simulink library "dspxfrm3"  (Simulink 8.3)
settings: Solver=ode45  SolverMode=SingleTasking  StartTime=0.0  StopTime=10.0  RelTol=1e-3
values from neighbouring files (symbols this model uses):
  D = D + B    [rebuffer_delay.m]
undefined symbols (not defined in the file or in its folder): dfilt, magnitude, Rows
libraries: dspsigops x6, dspxfrm3 x6, dspmtrx3 x6, dspsigattribs x5, dspmlti4 x2, dsparch4 x1, dspspect3 x1
settings Model: RequirementInfo=9  FPTRunName=Active  Creator=szlotkin  LastModifiedBy=apakyari  CovMetricSettings=d  ExtModeAutoUpdateStatusClock=off

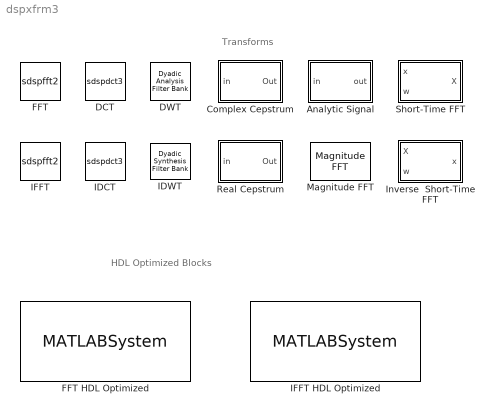
== system dspxfrm3 ==
  note: Transforms
  note: HDL Optimized Blocks
  Analytic Signal : Subsystem  mask(Analytic Signal){N=100, InputProcessing=Columns as channels (frame based)}
      mask prompts: N "Filter order (must be even):"; InputProcessing "Input processing:"
      mask help: Complex analytic signal of input.
      mask init:
      | x = [0,NaN,100,NaN,[58 58],NaN,[24 92],NaN,[58 24 24 58],NaN,[58 64 68 72 76 80 84 88],NaN, [42 42],NaN,[8 76],NaN,[72 68 64 60 56 52 48 42 36 32 28 24 20 16 12],NaN,[32 43 45 43 35]];
      | y = [0,NaN,100,NaN,[43 8],NaN,[16 16],NaN,[18 18 17 17],NaN,[16 24 36 24 28 28 32 16],NaN, [92 56],NaN,[64 64],NaN,[64 80 76 76 72 84 72 64 72 84 72 76 76 80 64],NaN,[51 33 41 33 35] ];
      | b=dspblkanalytic2('design',true,N);
      | dspblkanalytic2('setup',true,InputProcessing);
      mask Help: eval('blocksethelp');
      mask TypeOptions InputProcessing: Columns as channels (frame based) | Elements as channels (sample based) | Inherited (this choice will be removed - see release notes)
      mask Display: plot(x,y)
  Complex Cepstrum : Subsystem  mask(Complex Cepstrum){inheritFFT=on, N=64}
      mask prompts: inheritFFT "Inherit FFT length from input port dimensions"; N "FFT length:"
      mask help: Complex cepstrum of input signal. Input is modified to remove possible phase discontinuity at +/- pi radians.
      mask init:
      | dspblkceps('init');
      mask Help: eval('blocksethelp');
      mask Callback inheritFFT: dspblkceps
      mask Display: disp('Complex\n Cepstrum')
  DCT : S-Function  DialogController=dvDDGCreate  DialogControllerArgs=DataTag4  FunctionName=sdspdct3  Parameters=0, CompMethod,Dimension, 1, 0, 0, 0,1,outputMin,outputMax,dtInfo.firstCoeffMode,dtInfo.firstCoeffWordLength,dtInfo.firstCoeffFracLength,dtInfo.prodOutputMode,dtInfo.prodOutputWordLength,dtInfo.prodOutputFracLength,dtInfo.accumMode,dtInfo.accumWordLength,dtInfo.accumFracLength,dtInfo.outputMode,dtInfo.outputWordLength,dtInfo.outputFracLength,dtInfo.roundingMode,dtInfo.overflowMode  EnableBusSupport=on  mask(DCT){CompMethod=Table lookup, Dimension=0, TableOpt=Speed, BitRevOrder=off, SkipNorm=off, firstCoeffMode=Same word length as input, firstCoeffWordLength=16, firstCoeffFracLength=15, firstCoeffDataTypeStr=Inherit: Same word length as input, firstCoeffLastDataTypeStr=Inherit: Same word length as input, outputMode=Inherit via internal rule, outputWordLength=16, outputFracLength=15, outputDataTypeStr=Inherit: Inherit via internal rule, outputLastDataTypeStr=Inherit: Inherit via internal rule, outputMin=[], outputMax=[], accumMode=Inherit via internal rule, accumWordLength=32, accumFracLength=30, accumDataTypeStr=Inherit: Inherit via internal rule, accumLastDataTypeStr=Inherit: Inherit via internal rule, prodOutputMode=Inherit via internal rule, prodOutputWordLength=32, prodOutputFracLength=30, prodOutputDataTypeStr=Inherit: Inherit via internal rule, prodOutputLastDataTypeStr=Inherit: Inherit via internal rule, roundingMode=Floor, overflowMode=off, LockScale=off}
      mask prompts: CompMethod "Sine and cosine computation:"; TableOpt "Optimize twiddle table for:"; BitRevOrder "Output in bit-reversed order"; SkipNorm "Skip divide-by-two on butterfly outputs for fixed-point signals"; firstCoeffMode "Fixed-point sine table attributes:"; firstCoeffWordLength "Sine table word length:"; firstCoeffFracLength "Sine table fraction length:"; firstCoeffDataTypeStr "Sine table data type string:"; firstCoeffLastDataTypeStr "Last sine table data type string:"; outputMode "Fixed-point output attributes:"; outputWordLength "Output word length:"; outputFracLength "Output fraction length:"; outputDataTypeStr "Output data type string:"; outputLastDataTypeStr "Last output data type string:"; outputMin "Output minimum:"; outputMax "Output maximum:"; accumMode "Fixed-point accumulator attributes:"; accumWordLength "Accumulator word length:"; accumFracLength "Accumulator fraction length:"; accumDataTypeStr "Accum data type string:"; accumLastDataTypeStr "Last accum data type string:"; prodOutputMode "Fixed-point product output attributes:"; prodOutputWordLength "Product output word length:"; prodOutputFracLength "Product output fraction length:"; prodOutputDataTypeStr "ProdOutput data type string:"; prodOutputLastDataTypeStr "Last prodOutput data type string:"; roundingMode "Round integer calculations toward:"; overflowMode "Saturate on integer overflow"; LockScale "Lock scaling"
      mask help: Compute the discrete cosine transform (DCT) across the first dimension of the input. The first dimension of the input must have a power-of-two length.
      mask init:
      | Dimension = 1;
      | blkh   = gcbh;
      | dtRows = dspblkGetFFTDTRowInfo();
      | dtInfo = dspGetUDTFixptDataTypeInfo(blkh, dtRows, true);
      mask Help: eval('blocksethelp');
      mask TypeOptions CompMethod: Trigonometric fcn | Table lookup
      mask TypeOptions TableOpt: Speed | Memory
      mask TypeOptions firstCoeffMode: Same word length as input | Specify word length
      mask TypeOptions outputMode: Inherit via internal rule | Same as input | Binary point scaling | Slope and bias scaling
      mask TypeOptions accumMode: Inherit via internal rule | Same as product output | Same as input | Binary point scaling | Slope and bias scaling
      mask TypeOptions prodOutputMode: Inherit via internal rule | Same as input | Binary point scaling | Slope and bias scaling
      mask TypeOptions roundingMode: Ceiling | Convergent | Floor | Nearest | Round | Simplest | Zero
      mask Display: disp(' DCT')
  DWT : dspmlti4/Dyadic Analysis Filter Bank  Wname=User-defined  OrdRec_ordDec=[1 / 1]  Order=2  LPF="[0.0352   -0.0854   -0.1350   0.4599   0.8069   0.3327]"  HPF="[-0.3327    0.8069   -0.4599   -0.1350    0.0854    0.0352]"  NumLevels=2  tree=Symmetric  Output=Single port
  FFT : S-Function  DialogController=dspDDGCreate  DialogControllerArgs=DataTag5  FunctionName=sdspfft2  Parameters=0,2,TableOpt,1,BitRevOrder,0,SkipNorm,0,InheritFFTLength,FFTLength,WrapInput,1,outputMin,outputMax,RowConvenienceOn,plannerMethod,FFTImplementation,dtInfo.firstCoeffMode,dtInfo.firstCoeffWordLength,dtInfo.firstCoeffFracLength,dtInfo.prodOutputMode,dtInfo.prodOutputWordLength,dtInfo.prodOutputFracLength,dtInfo.accumMode,dtInfo.accumWordLength,dtInfo.accumFracLength,dtInfo.outputMode,dtInfo.outputWordLength,dtInfo.outputFracLength,dtInfo.roundingMode,dtInfo.overflowMode  EnableBusSupport=off  mask(FFT){CompMethod=Table lookup, TableOpt=NEW, TableOptActive=Speed, BitRevOrder=off, InheritFFTLength=on, FFTLength=64, WrapInput=on, RowConvenienceOn=on, FFTImplementation=Auto, additionalParams=off, SkipNorm=off, allowOverrides=on, firstCoeffMode=Same word length as input, firstCoeffWordLength=16, firstCoeffFracLength=15, firstCoeffDataTypeStr=Inherit: Same word length as input, firstCoeffLastDataTypeStr=Inherit: Same word length as input, outputMode=Inherit via internal rule, outputWordLength=16, outputFracLength=15, outputDataTypeStr=Inherit: Inherit via internal rule, outputLastDataTypeStr=Inherit: Inherit via internal rule, outputMin=[], outputMax=[], accumMode=Inherit via internal rule, accumWordLength=32, accumFracLength=30, accumDataTypeStr=Inherit: Inherit via internal rule, accumLastDataTypeStr=Inherit: Inherit via internal rule, prodOutputMode=Inherit via internal rule, prodOutputWordLength=32, prodOutputFracLength=30, prodOutputDataTypeStr=Inherit: Inherit via internal rule, prodOutputLastDataTypeStr=Inherit: Inherit via internal rule, roundingMode=Floor, overflowMode=off, LockScale=off}
      mask prompts: CompMethod "Twiddle factor computation:"; TableOpt "Optimize table for (obsolete):"; TableOptActive "Optimize table for:"; BitRevOrder "Output in bit-reversed order"; InheritFFTLength "Inherit FFT length from input dimensions"; FFTLength "FFT length:"; WrapInput "Wrap input data when FFT length is shorter than input length"; RowConvenienceOn "Perform row convenience"; FFTImplementation "FFT implementation:"; additionalParams "---------- Show additional parameters ----------"; SkipNorm "Skip divide-by-two on butterfly outputs for fixed-point signals"; allowOverrides "Allow overrides from DSP Fixed-Point Attributes blocks"; firstCoeffMode "Fixed-point sine table attributes:"; firstCoeffWordLength "Sine table word length:"; firstCoeffFracLength "Sine table fraction length:"; firstCoeffDataTypeStr "Sine table data type string:"; firstCoeffLastDataTypeStr "Last sine table data type string:"; outputMode "Fixed-point output attributes:"; outputWordLength "Output word length:"; outputFracLength "Output fraction length:"; outputDataTypeStr "Output data type string:"; outputLastDataTypeStr "Last output data type string:"; outputMin "Output minimum:"; outputMax "Output maximum:"; accumMode "Fixed-point accumulator attributes:"; accumWordLength "Accumulator word length:"; accumFracLength "Accumulator fraction length:"; accumDataTypeStr "Accum data type string:"; accumLastDataTypeStr "Last accum data type string:"; prodOutputMode "Fixed-point product output attributes:"; prodOutputWordLength "Product output word length:"; prodOutputFracLength "Product output fraction length:"; prodOutputDataTypeStr "ProdOutput data type string:"; prodOutputLastDataTypeStr "Last prodOutput data type string:"; roundingMode "Round integer calculations toward:"; overflowMode "Saturate on integer overflow"; LockScale "Lock scaling"
      mask help:
      | Compute the fast Fourier transform (FFT) across the first dimension of the input.
      |
      | When you set the 'FFT implementation' parameter to 'Radix-2', the FFT length must be a power of two.
      mask init:
      | blkh = gcbh;
      | plannerMethod = dspfftcontrol();
      | if ~(strcmp(get_param(blkh,'TableOpt'),'HYBRID') ||  strcmp(get_param(blkh,'TableOpt'),'NEW'))
      |   % this block lives in older version of SP BlockSet
      |     set_param(blkh,'TableOptActive',get_param(blkh,'TableOpt'));
      |     set_param(blkh,'TableOpt','HYBRID');
      |     if (strcmp(get_param(blkh,'SkipNorm'),'on'))
      |         set_param(blkh,'SkipNorm','off');
      |     else
      |         set_param(blkh,'SkipNorm','on');
      |     end
      | end
      | dtRows = dspblkGetFFTDTRowInfo();
      | dtInfo = dspGetUDTFixptDataTypeInfo(blkh, dtRows, true);
      mask Help: eval('blocksethelp');
      mask TypeOptions CompMethod: Trigonometric fcn | Table lookup
      mask TypeOptions TableOpt: Speed | Memory | HYBRID | NEW
      mask TypeOptions TableOptActive: Speed | Memory
      mask TypeOptions FFTImplementation: Auto | Radix-2 | FFTW
      mask TypeOptions firstCoeffMode: Same word length as input | Specify word length | Same as input | Same as output | User-defined | Binary point scaling | Slope and bias scaling
      mask TypeOptions outputMode: Inherit via internal rule | Same as input | Binary point scaling | Slope and bias scaling | User-defined
      mask TypeOptions accumMode: Inherit via internal rule | Same as product output | Same as input | Binary point scaling | Slope and bias scaling | User-defined
      mask TypeOptions prodOutputMode: Inherit via internal rule | Same as input | Binary point scaling | Slope and bias scaling | User-defined
      mask TypeOptions roundingMode: Ceiling | Convergent | Floor | Nearest | Round | Simplest | Zero
      mask Display: disp('  FFT ');
  FFT HDL Optimized : MATLABSystem  System=dsp.HDLFFT  Normalize=off  FFTLengthSource=Property  FFTLength=1024  RoundingMethod=Floor  OverflowAction=Wrap  ValidInputPort=on  StartOutputPort=off  EndOutputPort=off
      mask Type: dsp.HDLFFT
      mask Display:
      | disp(['FFT' char(10) 'HDL Optimized' char(10) 'Latency, 1589']);
      | port_label('input',1,'dataIn');
      | port_label('input',2,'validIn');
      | port_label('output',1,'dataOut');
      | port_label('output',2,'validOut');
  IDCT : S-Function  DialogController=dvDDGCreate  DialogControllerArgs=DataTag6  FunctionName=sdspdct3  Parameters=1,CompMethodActive, Dimension, 1, 0, 0, 0,outSamplingMode,outputMin,outputMax,dtInfo.firstCoeffMode,dtInfo.firstCoeffWordLength,dtInfo.firstCoeffFracLength,dtInfo.prodOutputMode,dtInfo.prodOutputWordLength,dtInfo.prodOutputFracLength,dtInfo.accumMode,dtInfo.accumWordLength,dtInfo.accumFracLength,dtInfo.outputMode,dtInfo.outputWordLength,dtInfo.outputFracLength,dtInfo.roundingMode,dtInfo.overflowMode  EnableBusSupport=on  mask(IDCT){CompMethod=HYBRID, CompMethodActive=Table lookup, Dimension=0, TableOpt=Speed, BitRevOrder=off, outSamplingMode=Sample based, SkipNorm=off, firstCoeffMode=Same word length as input, firstCoeffWordLength=16, firstCoeffFracLength=15, firstCoeffDataTypeStr=Inherit: Same word length as input, firstCoeffLastDataTypeStr=Inherit: Same word length as input, outputMode=Inherit via internal rule, outputWordLength=16, outputFracLength=15, outputDataTypeStr=Inherit: Inherit via internal rule, outputLastDataTypeStr=Inherit: Inherit via internal rule, outputMin=[], outputMax=[], accumMode=Inherit via internal rule, accumWordLength=32, accumFracLength=30, accumDataTypeStr=Inherit: Inherit via internal rule, accumLastDataTypeStr=Inherit: Inherit via internal rule, prodOutputMode=Inherit via internal rule, prodOutputWordLength=32, prodOutputFracLength=30, prodOutputDataTypeStr=Inherit: Inherit via internal rule, prodOutputLastDataTypeStr=Inherit: Inherit via internal rule, roundingMode=Floor, overflowMode=off, LockScale=off}
      mask prompts: CompMethod "Twiddle factor computation obsolete:"; CompMethodActive "Sine and cosine computation:"; TableOpt "Optimize twiddle table for:"; BitRevOrder "Output in bit-reversed order"; outSamplingMode "OUtput sampling mode"; SkipNorm "Skip divide-by-two on butterfly outputs for fixed-point signals"; firstCoeffMode "Fixed-point sine table attributes:"; firstCoeffWordLength "Sine table word length:"; firstCoeffFracLength "Sine table fraction length:"; firstCoeffDataTypeStr "Sine table data type string:"; firstCoeffLastDataTypeStr "Last sine table data type string:"; outputMode "Fixed-point output attributes:"; outputWordLength "Output word length:"; outputFracLength "Output fraction length:"; outputDataTypeStr "Output data type string:"; outputLastDataTypeStr "Last output data type string:"; outputMin "Output minimum:"; outputMax "Output maximum:"; accumMode "Fixed-point accumulator attributes:"; accumWordLength "Accumulator word length:"; accumFracLength "Accumulator fraction length:"; accumDataTypeStr "Accum data type string:"; accumLastDataTypeStr "Last accum data type string:"; prodOutputMode "Fixed-point product output attributes:"; prodOutputWordLength "Product output word length:"; prodOutputFracLength "Product output fraction length:"; prodOutputDataTypeStr "ProdOutput data type string:"; prodOutputLastDataTypeStr "Last prodOutput data type string:"; roundingMode "Round integer calculations toward:"; overflowMode "Saturate on integer overflow"; LockScale "Lock scaling"
      mask help: Compute the inverse discrete cosine transform (IDCT) across the first dimension of the input. The first dimension of the input must have a power-of-two length.
      mask init:
      | Dimension = 1;
      | blkh      = gcbh;
      | if ~(strcmp(get_param(blkh,'CompMethod'),'HYBRID') ||  strcmp(get_param(blkh,'CompMethod'),'NEW'))
      |   % this block lives in older version of SP BlockSet
      |     set_param(blkh,'outSamplingMode','Frame based');
      |     set_param(blkh,'CompMethodActive',get_param(blkh,'CompMethod'));
      |     set_param(blkh,'CompMethod','HYBRID');
      | end
      | dtRows = dspblkGetFFTDTRowInfo();
      | dtInfo = dspGetUDTFixptDataTypeInfo(blkh, dtRows, true);
      mask Help: eval('blocksethelp');
      mask TypeOptions CompMethod: Trigonometric fcn | Table lookup | HYBRID | NEW
      mask TypeOptions CompMethodActive: Trigonometric fcn | Table lookup
      mask TypeOptions TableOpt: Speed | Memory
      mask TypeOptions outSamplingMode: Sample based | Frame based
      mask TypeOptions firstCoeffMode: Same word length as input | Specify word length
      mask TypeOptions outputMode: Inherit via internal rule | Same as input | Binary point scaling | Slope and bias scaling
      mask TypeOptions accumMode: Inherit via internal rule | Same as product output | Same as input | Binary point scaling | Slope and bias scaling
      mask TypeOptions prodOutputMode: Inherit via internal rule | Same as input | Binary point scaling | Slope and bias scaling
      mask TypeOptions roundingMode: Ceiling | Convergent | Floor | Nearest | Round | Simplest | Zero
      mask Display: disp('IDCT')
  IDWT : dspmlti4/Dyadic Synthesis Filter Bank  Wname=User-defined  OrdRec_ordDec=[1 / 1]  Order=2  LPF="[0.3327    0.8069    0.4599   -0.1350   -0.0854    0.0352]"  HPF="[0.0352    0.0854   -0.1350   -0.4599    0.8069   -0.3327]"  NumLevels=2  tree=Symmetric  Input=Single port
  IFFT : S-Function  DialogController=dspDDGCreate  DialogControllerArgs=DataTag7  FunctionName=sdspfft2  Parameters=1,2,TableOpt,1,BitRevOrder,cs_in,SkipNorm,0,InheritFFTLength,FFTLength,WrapInput,outSamplingMode,outputMin,outputMax,RowConvenienceOn,plannerMethod,FFTImplementation,dtInfo.firstCoeffMode,dtInfo.firstCoeffWordLength,dtInfo.firstCoeffFracLength,dtInfo.prodOutputMode,dtInfo.prodOutputWordLength,dtInfo.prodOutputFracLength,dtInfo.accumMode,dtInfo.accumWordLength,dtInfo.accumFracLength,dtInfo.outputMode,dtInfo.outputWordLength,dtInfo.outputFracLength,dtInfo.roundingMode,dtInfo.overflowMode  EnableBusSupport=off  mask(IFFT){CompMethod=Table lookup, TableOpt=NEW, TableOptActive=Speed, BitRevOrder=off, cs_in=off, SkipNorm=on, InheritFFTLength=on, FFTLength=64, WrapInput=on, mode=Complex, outSamplingMode=Sample based, RowConvenienceOn=on, FFTImplementation=Auto, additionalParams=off, allowOverrides=on, firstCoeffMode=Same word length as input, firstCoeffWordLength=16, firstCoeffFracLength=15, firstCoeffDataTypeStr=Inherit: Same word length as input, firstCoeffLastDataTypeStr=Inherit: Same word length as input, outputMode=Inherit via internal rule, outputWordLength=16, outputFracLength=15, outputDataTypeStr=Inherit: Inherit via internal rule, outputLastDataTypeStr=Inherit: Inherit via internal rule, outputMin=[], outputMax=[], accumMode=Inherit via internal rule, accumWordLength=32, accumFracLength=30, accumDataTypeStr=Inherit: Inherit via internal rule, accumLastDataTypeStr=Inherit: Inherit via internal rule, prodOutputMode=Inherit via internal rule, prodOutputWordLength=32, prodOutputFracLength=30, prodOutputDataTypeStr=Inherit: Inherit via internal rule, prodOutputLastDataTypeStr=Inherit: Inherit via internal rule, roundingMode=Floor, overflowMode=off, LockScale=off}
      mask prompts: CompMethod "Twiddle factor computation:"; TableOpt "Optimize table for (obsolete):"; TableOptActive "Optimize table for:"; BitRevOrder "Input is in bit-reversed order"; cs_in "Input is conjugate symmetric"; SkipNorm "Skip scaling"; InheritFFTLength "Inherit FFT length from input dimensions"; FFTLength "FFT length:"; WrapInput "Wrap input data when FFT length is shorter than input length"; mode "Output:"; outSamplingMode "OUtput sampling mode"; RowConvenienceOn "Perform row convenience"; FFTImplementation "FFT implementation:"; additionalParams "---------- Show additional parameters ----------"; allowOverrides "Allow overrides from DSP FPA Fixed-Point Attributes blocks"; firstCoeffMode "Fixed-point sine table attributes:"; firstCoeffWordLength "Sine table word length:"; firstCoeffFracLength "Sine table fraction length:"; firstCoeffDataTypeStr "Sine table data type string:"; firstCoeffLastDataTypeStr "Last sine table data type string:"; outputMode "Fixed-point output attributes:"; outputWordLength "Output word length:"; outputFracLength "Output fraction length:"; outputDataTypeStr "Output data type string:"; outputLastDataTypeStr "Last output data type string:"; outputMin "Output minimum:"; outputMax "Output maximum:"; accumMode "Fixed-point accumulator attributes:"; accumWordLength "Accumulator word length:"; accumFracLength "Accumulator fraction length:"; accumDataTypeStr "Accum data type string:"; accumLastDataTypeStr "Last accum data type string:"; prodOutputMode "Fixed-point product output attributes:"; prodOutputWordLength "Product output word length:"; prodOutputFracLength "Product output fraction length:"; prodOutputDataTypeStr "ProdOutput data type string:"; prodOutputLastDataTypeStr "Last prodOutput data type string:"; roundingMode "Round integer calculations toward:"; overflowMode "Saturate on integer overflow"; LockScale "Lock scaling"
      mask help:
      | Compute the inverse fast Fourier transform (IFFT) across the first dimension of the input.
      |
      | When you set the 'FFT implementation' parameter to 'Radix-2', the FFT length must be a power of two.
      mask init:
      | blkh = gcbh;
      | plannerMethod = dspfftcontrol();
      | if ~(strcmp(get_param(blkh,'TableOpt'),'HYBRID') ||  strcmp(get_param(blkh,'TableOpt'),'NEW'))
      |   % this block lives in older version of SP BlockSet
      | %     set_param(blkh,'frameSpecViaDialog','off');
      |     set_param(blkh,'outSamplingMode','Frame based');
      |     set_param(blkh,'TableOptActive',get_param(blkh,'TableOpt'));
      |     set_param(blkh,'TableOpt','HYBRID');
      |     if (strcmp(get_param(blkh,'SkipNorm'),'on'))
      |         set_param(blkh,'SkipNorm','off');
      |     else
      |         set_param(blkh,'SkipNorm','on');
      |     end    
      | end
      | dtRows = dspblkGetFFTDTRowInfo();
      | dtInfo = dspGetUDTFixptDataTypeInfo(blkh, dtRows, true);
      mask Help: eval('blocksethelp');
      mask TypeOptions CompMethod: Trigonometric fcn | Table lookup
      mask TypeOptions TableOpt: Speed | Memory | HYBRID | NEW
      mask TypeOptions TableOptActive: Speed | Memory
      mask TypeOptions mode: Real | Complex
      mask TypeOptions outSamplingMode: Sample based | Frame based
      mask TypeOptions FFTImplementation: Auto | Radix-2 | FFTW
      mask TypeOptions firstCoeffMode: Same word length as input | Specify word length | Same as input | Same as output | User-defined | Binary point scaling | Slope and bias scaling
      mask TypeOptions outputMode: Inherit via internal rule | Same as input | Binary point scaling | Slope and bias scaling | User-defined
      mask TypeOptions accumMode: Inherit via internal rule | Same as product output | Same as input | Binary point scaling | Slope and bias scaling | User-defined
      mask TypeOptions prodOutputMode: Inherit via internal rule | Same as input | Binary point scaling | Slope and bias scaling | User-defined
      mask TypeOptions roundingMode: Ceiling | Convergent | Floor | Nearest | Round | Simplest | Zero
      mask Display: disp('  IFFT')
  IFFT HDL Optimized : MATLABSystem  System=dsp.HDLIFFT  Normalize=on  FFTLengthSource=Property  FFTLength=1024  RoundingMethod=Floor  OverflowAction=Wrap  ValidInputPort=on  StartOutputPort=off  EndOutputPort=off
      mask Type: dsp.HDLIFFT
      mask Display:
      | disp(['IFFT' char(10) 'HDL Optimized' char(10) 'Latency, 1589']);
      | port_label('input',1,'dataIn');
      | port_label('input',2,'validIn');
      | port_label('output',1,'dataOut');
      | port_label('output',2,'validOut');
  Inverse  Short-Time FFT : Subsystem  mask(Inverse Short-Time FFT){W=512, OvLap=384, OutFrameSize=512, InConjSymm=on, DoAssert=off, Tol=1e-4}
      mask prompts: W "Analysis window length:"; OvLap "Overlap between consecutive STFFT frames (in samples):"; OutFrameSize "Samples per output frame:"; InConjSymm "Input is conjugate symmetric"; DoAssert "Assert if analysis window does not support perfect signal reconstruction"; Tol "Reconstruction error tolerance:"
      mask help:
      | Reconstructs a signal from its Short-Time FFT (STFFT) by using the OLA method. The block takes as an input the analysis window w[n] used in the generation of the STFFT to normalize the output signal.
      |
      | Optionally, the block asserts if the analysis window does not satisfy constraints that permit perfect reconstruction of the signal.
      mask init:
      | L = dspblkistfft('init',DoAssert,OvLap,W,InConjSymm);
      mask Help: eval('blocksethelp');
      mask Callback DoAssert: dspblkistfft('dynamic');
      mask Display:
      | port_label('input',1,'X[nL,k]')
      | port_label('output',1,'x[n]')
      | port_label('input',2,'w[n]')
  Magnitude FFT : dspspect3/Magnitude FFT  mag_or_magsq=Magnitude squared  FFTImplementation=Auto  fftLenInherit=off  fftsize=256  WrapInput=on
  Real Cepstrum : Subsystem  mask(Real Cepstrum){inheritFFT=on, N=64}
      mask prompts: inheritFFT "Inherit FFT length from input port dimensions"; N "FFT length:"
      mask help: Real cepstrum of input signal.
      mask init:
      | dspblkceps('init');
      mask Help: eval('blocksethelp');
      mask Callback inheritFFT: dspblkceps
      mask Display: disp('Real\nCepstrum')
  Short-Time FFT : Subsystem  mask(Short-Time FFT){W=512, OvLap=384, M=1024, TreatMby1Signals=One channel}
      mask prompts: W "Analysis window length:"; OvLap "Overlap between consecutive windows (in samples):"; M "FFT length:"; TreatMby1Signals "Treat Mx1 and unoriented sample-based signals as:"
      mask help:
      | Output the Short-Time FFT of the input signal x[n].
      | Uses an externally specified analysis window w[n].
      mask init:
      | dspSetFrameUpgradeParameter(gcbh, 'TreatMby1Signals', 'M channels (this choice will be removed - see release notes)');
      | 
      | if W == 1
      |     error('spblockset:ShortTimeFFT:winLenOne', ...
      |           'The analysis window length must be greater than 1');
      | end
      | 
      | L = W-OvLap;
      | BufferBlkName = [gcb '/Rebuffer'];
      | set_param(BufferBlkName, 'TreatMby1Signals', ...
      |           get_param(gcb, 'TreatMby1Signals'));
      mask Help: eval('blocksethelp');
      mask TypeOptions TreatMby1Signals: One channel | M channels (this choice will be removed - see release notes)
      mask Display:
      | port_label('input',1,'x[n]')
      | port_label('input',2,'w[n]')
      | port_label('output',1,'X[nL,k]')

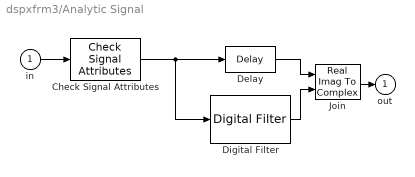
== system dspxfrm3/Analytic Signal ==
  in : Inport
  Check Signal Attributes : dspsigattribs/Check Signal Attributes  SystemSampleTime=-1  SigAttribCheckMethod=Does not match attributes exactly  Complexity=Ignore  Frame=Ignore  DimsCheckMethod=Ignore  Dimensions=1-D  DatatypeCheckMethod=Is...  DatatypeGeneral=Floating-point  DtypeFloatSpecific=Any floating-point  DtypeFixedSpecific=Any fixed-point  DtypeIntSpecific=Any integer  SampleMode=Ignore
  Delay : dspsigops/Delay  InputProcessing=Columns as channels (frame based)  dly_unit=Samples  delay=N/2  ic_detail=off  dif_ic_for_ch=off  dif_ic_for_dly=off  ic=0  reset_popup=None
  Digital Filter : dsparch4/Digital Filter  TypePopup=FIR (all zeros)  IIRFiltStruct=Direct form II transposed  AllPoleFiltStruct=Direct form  FIRFiltStruct=Direct form transposed  CoeffSource=Specify via dialog  NumCoeffs=b  DenCoeffs=[1 0.1]  BiQuadCoeffs=[1 0.3 0.4 1 0.1 0.2]  LatticeCoeffs=[0.2 0.4]  denIgnore=on  FiltPerSampPopup=One filter per frame  IC=0  ICnum=0  ICden=0  roundingMode=Floor  overflowMode=off  ScaleValues=1  scaleValueFracLength=14  stageInFracLength=15  stageOutFracLength=15  FilterSource=Specify via dialog  dfiltObjectName=dfilt.dffir([1 2 1])  InputProcessing=Columns as channels (frame based)
  Join : RealImagToComplex
  out : Outport  InitialOutput=0
  wires:
  Check Signal Attributes/1 -> Digital Filter/1, Delay/1
  in/1 -> Check Signal Attributes/1
  Join/1 -> out/1
  Delay/1 -> Join/1
  Digital Filter/1 -> Join/2

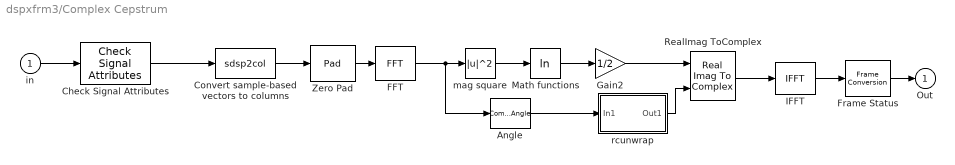
== system dspxfrm3/Complex Cepstrum ==
  in : Inport
  Angle : ComplexToMagnitudeAngle  Output=Angle
  Check Signal Attributes : dspsigattribs/Check Signal Attributes  SigAttribCheckMethod=Does not match attributes exactly  Complexity=Real  Frame=Ignore  DimsCheckMethod=Ignore  Dimensions=1-D  DatatypeCheckMethod=Is...  DatatypeGeneral=Floating-point  DtypeFloatSpecific=Any floating-point  DtypeFixedSpecific=Any fixed-point  DtypeIntSpecific=Any integer  SampleMode=Discrete
  Convert sample-based vectors to columns : S-Function  FunctionName=sdsp2col  EnableBusSupport=off
  FFT : dspxfrm3/FFT  CompMethod=Table lookup  TableOpt=NEW  TableOptActive=Speed  BitRevOrder=off  InheritFFTLength=on  FFTLength=64  RowConvenienceOn=on  FFTImplementation=Auto  SkipNorm=off  firstCoeffDataTypeStr=Inherit: Same word length as input  firstCoeffLastDataTypeStr=Inherit: Same word length as input  outputMin=[]  outputMax=[]  roundingMode=Floor  overflowMode=off
  Frame Status : FrameConversion  OutFrame=Sample-based
  Gain2 : Gain  Gain=1/2  SaturateOnIntegerOverflow=on  OutDataTypeStr=Inherit: Same as input  ParamDataTypeStr=Inherit: Same as input
  IFFT : dspxfrm3/IFFT  CompMethod=Table lookup  TableOpt=HYBRID  TableOptActive=Speed  BitRevOrder=off  cs_in=on  SkipNorm=on  InheritFFTLength=on  FFTLength=64  mode=Real  outSamplingMode=Frame based  RowConvenienceOn=on  FFTImplementation=Auto  firstCoeffDataTypeStr=Inherit: Same word length as input  firstCoeffLastDataTypeStr=Inherit: Same word length as input  outputMin=[]  outputMax=[]  roundingMode=Floor  overflowMode=off
  Math functions : Math  Operator=log  SaturateOnIntegerOverflow=on
  RealImag ToComplex : RealImagToComplex
  Zero Pad : dspsigops/Pad  padAlong=None  dimsToPad=1  valSrc=Specify via dialog  padVal=0  spec=Output size  padNumOutRowsSpecMethod=User-specified  numOutRows=N  padNumOutColsSpecMethod=User-specified  numOutCols=1  isVarDimsMode=off  padBeginning=0  padEnd=0  outSizeMode=User-specified  outSize=1  padSigAt=End  trunc_flag=None  roundingMode=Floor  overflowMode=off  truncOrWrapMode=Truncate  wrap_flag=None
  mag square : Math  Operator=magnitude^2  SaturateOnIntegerOverflow=on
  rcunwrap : Subsystem
  Out : Outport  InitialOutput=0
  wires:
  Check Signal Attributes/1 -> Convert sample-based vectors to columns/1
  RealImag ToComplex/1 -> IFFT/1
  Frame Status/1 -> Out/1
  Zero Pad/1 -> FFT/1
  Convert sample-based vectors to columns/1 -> Zero Pad/1
  IFFT/1 -> Frame Status/1
  Angle/1 -> rcunwrap/1(In1)
  FFT/1 -> Angle/1, mag square/1
  in/1 -> Check Signal Attributes/1
  Math functions/1 -> Gain2/1
  mag square/1 -> Math functions/1
  rcunwrap/1(Out1) -> RealImag ToComplex/2
  Gain2/1 -> RealImag ToComplex/1

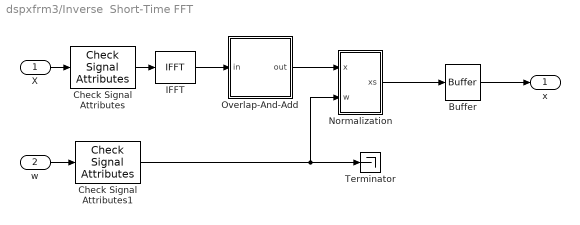
== system dspxfrm3/Inverse  Short-Time FFT ==
  X : Inport
  w : Inport  Port=2
  Buffer : Buffer  N=OutFrameSize  TreatMby1Signals=One channel
  Check Signal Attributes : dspsigattribs/Check Signal Attributes  SigAttribCheckMethod=Does not match attributes exactly  Complexity=Ignore  Frame=Ignore  DimsCheckMethod=Ignore  Dimensions=1-D  DatatypeCheckMethod=Is...  DatatypeGeneral=Floating-point  DtypeFloatSpecific=Any floating-point  DtypeFixedSpecific=Any fixed-point  DtypeIntSpecific=Any integer  SampleMode=Ignore
  Check Signal Attributes1 : dspsigattribs/Check Signal Attributes  SigAttribCheckMethod=Does not match attributes exactly  Complexity=Ignore  Frame=Ignore  DimsCheckMethod=Ignore  Dimensions=1-D  DatatypeCheckMethod=Is...  DatatypeGeneral=Floating-point  DtypeFloatSpecific=Any floating-point  DtypeFixedSpecific=Any fixed-point  DtypeIntSpecific=Any integer  SampleMode=Ignore
  IFFT : dspxfrm3/IFFT  CompMethod=Table lookup  TableOpt=HYBRID  TableOptActive=Speed  BitRevOrder=off  cs_in=on  SkipNorm=on  InheritFFTLength=on  FFTLength=64  WrapInput=on  mode=Real  outSamplingMode=Frame based  RowConvenienceOn=on  FFTImplementation=Auto  firstCoeffDataTypeStr=Inherit: Same word length as input  firstCoeffLastDataTypeStr=Inherit: Same word length as input  outputMin=[]  outputMax=[]  roundingMode=Floor  overflowMode=off
  Normalization : Subsystem
  Overlap-And-Add : Subsystem  mask(Overlap-And-Add){L=L}
      mask prompts: L "Number of new points in each frame"
      mask help: Performs overlap-and-add on the input signal. Disjoint frames of the input signal are overlapped with each other for a specified number of points and summed.
      mask Display: disp('Overlap\nAnd\nAdd')
  Terminator : Terminator
  x : Outport
  wires:
  Check Signal Attributes1/1 -> Terminator/1, Normalization/2(w)
  Check Signal Attributes/1 -> IFFT/1
  Buffer/1 -> x/1
  w/1 -> Check Signal Attributes1/1
  X/1 -> Check Signal Attributes/1
  Overlap-And-Add/1(out) -> Normalization/1(x)
  IFFT/1 -> Overlap-And-Add/1(in)
  Normalization/1(xs) -> Buffer/1

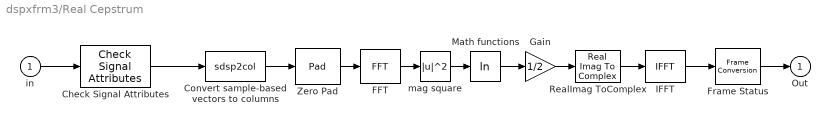
== system dspxfrm3/Real Cepstrum ==
  in : Inport
  Check Signal Attributes : dspsigattribs/Check Signal Attributes  SystemSampleTime=-1  SigAttribCheckMethod=Does not match attributes exactly  Complexity=Real  Frame=Ignore  DimsCheckMethod=Ignore  Dimensions=1-D  DatatypeCheckMethod=Is...  DatatypeGeneral=Floating-point  DtypeFloatSpecific=Any floating-point  DtypeFixedSpecific=Any fixed-point  DtypeIntSpecific=Any integer  SampleMode=Discrete
  Convert sample-based vectors to columns : S-Function  FunctionName=sdsp2col  EnableBusSupport=off
  FFT : dspxfrm3/FFT  CompMethod=Table lookup  TableOpt=NEW  TableOptActive=Speed  BitRevOrder=off  InheritFFTLength=on  FFTLength=64  SkipNorm=off  roundingMode=Floor  overflowMode=off
  Frame Status : FrameConversion  OutFrame=Sample-based
  Gain : Gain  Gain=1/2  SaturateOnIntegerOverflow=on  OutDataTypeStr=Inherit: Same as input  ParamDataTypeStr=Inherit: Same as input
  IFFT : dspxfrm3/IFFT  CompMethod=Table lookup  TableOpt=HYBRID  TableOptActive=Speed  BitRevOrder=off  cs_in=on  SkipNorm=on  InheritFFTLength=on  FFTLength=64  mode=Real  outSamplingMode=Frame based  roundingMode=Floor  overflowMode=off
  Math functions : Math  Operator=log  SaturateOnIntegerOverflow=on
  RealImag ToComplex : RealImagToComplex  Input=Real
  Zero Pad : dspsigops/Pad  padAlong=None  dimsToPad=1  valSrc=Specify via dialog  padVal=0  spec=Output size  padNumOutRowsSpecMethod=User-specified  numOutRows=N  padNumOutColsSpecMethod=User-specified  numOutCols=1  isVarDimsMode=off  padBeginning=0  padEnd=0  outSizeMode=User-specified  outSize=1  padSigAt=End  trunc_flag=None  roundingMode=Floor  overflowMode=off  truncOrWrapMode=Truncate  wrap_flag=None
  mag square : Math  Operator=magnitude^2  SaturateOnIntegerOverflow=on
  Out : Outport  InitialOutput=0
  wires:
  Check Signal Attributes/1 -> Convert sample-based vectors to columns/1
  RealImag ToComplex/1 -> IFFT/1
  Frame Status/1 -> Out/1
  Convert sample-based vectors to columns/1 -> Zero Pad/1
  IFFT/1 -> Frame Status/1
  Gain/1 -> RealImag ToComplex/1
  Math functions/1 -> Gain/1
  mag square/1 -> Math functions/1
  FFT/1 -> mag square/1
  in/1 -> Check Signal Attributes/1
  Zero Pad/1 -> FFT/1

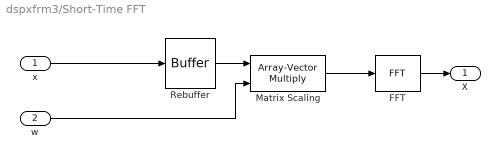
== system dspxfrm3/Short-Time FFT ==
  x : Inport
  w : Inport  Port=2
  FFT : dspxfrm3/FFT  CompMethod=Table lookup  TableOpt=NEW  TableOptActive=Speed  BitRevOrder=off  InheritFFTLength=off  FFTLength=M  RowConvenienceOn=off  SkipNorm=off  firstCoeffDataTypeStr=Inherit: Same word length as input  firstCoeffLastDataTypeStr=Inherit: Same word length as input  outputMin=[]  outputMax=[]  roundingMode=Floor  overflowMode=off
  Matrix Scaling : dspmtrx3/Array-Vector Multiply  mode=Mute  saveAsFlag=0  Dimension=1  V_Source=Input port  V_VectFromMask=[0.5 0.25]  firstCoeffSignedness=Auto  firstCoeffDataTypeStr=Inherit: Same word length as input  firstCoeffLastDataTypeStr=Inherit: Same word length as input  firstCoeffMin=[]  firstCoeffMax=[]  outputSignedness=Auto  outputMin=[]  outputMax=[]  accumSignedness=Auto  prodOutputSignedness=Auto  roundingMode=Floor  overflowMode=off
  Rebuffer : Buffer  N=W  V=W-L  TreatMby1Signals=One channel
  X : Outport
  wires:
  Matrix Scaling/1 -> FFT/1
  Rebuffer/1 -> Matrix Scaling/1
  x/1 -> Rebuffer/1
  w/1 -> Matrix Scaling/2
  FFT/1 -> X/1

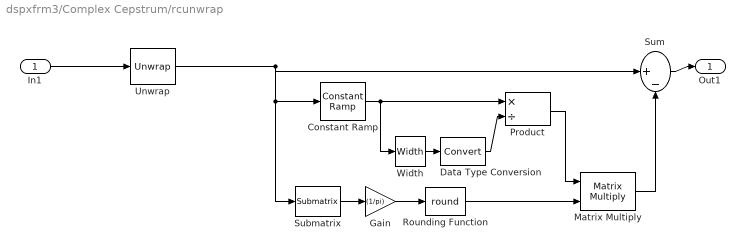
== system dspxfrm3/Complex Cepstrum/rcunwrap ==
  In1 : Inport
  Constant Ramp : dspsigops/Constant Ramp  L=Rows  dim=1  Slope=2*pi  dataType=Same as input  isSigned=on  wordLen=16  udDataType=sfix(16)  fracBitsMode=Best precision  numFracBits=15  Offset=0
  Data Type Conversion : DataTypeConversion  SaturateOnIntegerOverflow=on  RndMeth=Zero
  Gain : Gain  Gain=(1/pi)  SaturateOnIntegerOverflow=on  OutDataTypeStr=Inherit: Same as input  ParamDataTypeStr=Inherit: Same as input
  Matrix Multiply : Product  Multiplication=Matrix(*)
  Product : Product  Inputs=*/  SaturateOnIntegerOverflow=on  InputSameDT=on  OutDataTypeStr=Inherit: Same as first input
  Rounding Function : Rounding  Operator=round
  Submatrix : dspmtrx3/Submatrix  RowSpan=One row  RowStartMode=Middle  RowStartIndex=1  RowEndMode=Last  RowEndIndex=1  ColSpan=All columns  ColStartMode=First  ColStartIndex=1  ColEndMode=Last  ColEndIndex=1
  Sum : Sum  Inputs=|+-  SaturateOnIntegerOverflow=on  InputSameDT=on  OutDataTypeStr=Inherit: Same as first input
  Unwrap : dspsigops/Unwrap  tol=pi  InputProcessing=Columns as channels (frame based)  running=on
  Width : Width  DataType=int32
  Out1 : Outport
  wires:
  Width/1 -> Data Type Conversion/1
  Data Type Conversion/1 -> Product/2
  Product/1 -> Matrix Multiply/1
  Constant Ramp/1 -> Width/1, Product/1
  Matrix Multiply/1 -> Sum/2
  Unwrap/1 -> Submatrix/1, Constant Ramp/1, Sum/1
  Submatrix/1 -> Gain/1
  Gain/1 -> Rounding Function/1
  Rounding Function/1 -> Matrix Multiply/2
  Sum/1 -> Out1/1
  In1/1 -> Unwrap/1

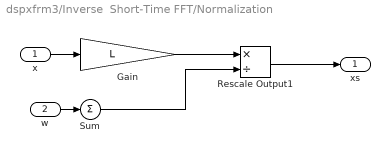
== system dspxfrm3/Inverse  Short-Time FFT/Normalization ==
  x : Inport
  w : Inport  Port=2
  Gain : Gain  Gain=L  SaturateOnIntegerOverflow=on  OutDataTypeStr=Inherit: Same as input  ParamDataTypeStr=Inherit: Same as input
  Rescale Output1 : Product  Inputs=*/  InputSameDT=on  OutDataTypeStr=Inherit: Same as first input
  Sum : Sum  Inputs=+  SaturateOnIntegerOverflow=on
  xs : Outport
  wires:
  x/1 -> Gain/1
  Rescale Output1/1 -> xs/1
  w/1 -> Sum/1
  Sum/1 -> Rescale Output1/2
  Gain/1 -> Rescale Output1/1

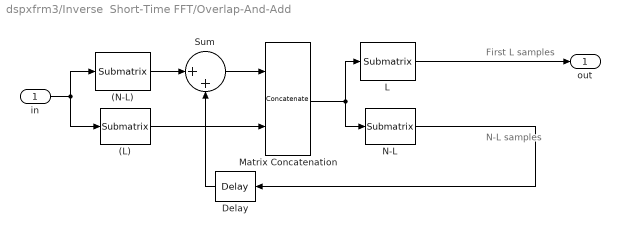
== system dspxfrm3/Inverse  Short-Time FFT/Overlap-And-Add ==
  note: First L samples
  note: N-L samples
  in : Inport
  (L) : dspmtrx3/Submatrix  RowSpan=Range of rows  RowStartMode=Offset from last  RowStartIndex=L-1  RowEndMode=Last  RowEndIndex=1  ColSpan=All columns  ColStartMode=First  ColStartIndex=1  ColEndMode=Last  ColEndIndex=1
  (N-L) : dspmtrx3/Submatrix  RowSpan=Range of rows  RowStartMode=First  RowStartIndex=1  RowEndMode=Offset from last  RowEndIndex=L  ColSpan=All columns  ColStartMode=First  ColStartIndex=1  ColEndMode=Last  ColEndIndex=1
  Delay : dspsigops/Delay  InputProcessing=Columns as channels (frame based)  dly_unit=Frames  delay=1  ic_detail=off  dif_ic_for_ch=off  dif_ic_for_dly=off  ic=0  reset_popup=None
  L : dspmtrx3/Submatrix  RowSpan=Range of rows  RowStartMode=First  RowStartIndex=1  RowEndMode=Index  RowEndIndex=L  ColSpan=All columns  ColStartMode=First  ColStartIndex=1  ColEndMode=Last  ColEndIndex=1
  Matrix Concatenation : Concatenate  Mode=Multidimensional array
  N-L : dspmtrx3/Submatrix  RowSpan=Range of rows  RowStartMode=Index  RowStartIndex=L+1  RowEndMode=Last  RowEndIndex=1  ColSpan=All columns  ColStartMode=First  ColStartIndex=1  ColEndMode=Last  ColEndIndex=1
  Sum : Sum  Inputs=|++  SaturateOnIntegerOverflow=on  InputSameDT=on  OutDataTypeStr=Inherit: Same as first input
  out : Outport
  wires:
  L/1 -> out/1
  Sum/1 -> Matrix Concatenation/1
  (N-L)/1 -> Sum/1
  Delay/1 -> Sum/2
  (L)/1 -> Matrix Concatenation/2
  N-L/1 -> Delay/1
  Matrix Concatenation/1 -> L/1, N-L/1
  in/1 -> (L)/1, (N-L)/1
